simulink model "Rec3_P3_TwoLinkArm"  (R2024b)
settings: Solver=VariableStepAuto  StartTime=0.0  StopTime=10.0  RelTol=1e-3
values from neighbouring files (symbols this model uses):
  A = (1-f)/0.005    (= 50)    [Rec3_P3_TwoLinkArm_Triangle_script.m]    (also in Rec_5_main.m)
  f = 0.75    [Rec3_P3_TwoLinkArm_Triangle_script.m]    (also in Rec_5_main.m)
  Kd1 = 1.6169    [Rec3_P3_TwoLinkArm_Triangle_script.m]    (also in Rec_5_main.m)
  Kd2 = Kd1    (= 1.6169)    [Rec3_P3_TwoLinkArm_Triangle_script.m]    (also in Rec_5_main.m)
  Kp1 = 11.4196    [Rec3_P3_TwoLinkArm_Triangle_script.m]    (also in Rec_5_main.m)
  Kp2 = Kp1    (= 11.4196)    [Rec3_P3_TwoLinkArm_Triangle_script.m]    (also in Rec_5_main.m)
  sim_t = [linspace(0,8,4*n)]    [Rec3_P3_TwoLinkArm_Triangle_script.m]
  theta_1_sim = zeros(1,length(sim_t))    [Rec3_P3_TwoLinkArm_Triangle_script.m]
  theta_2_sim = zeros(1,length(sim_t))    [Rec3_P3_TwoLinkArm_Triangle_script.m]
settings Model: Creator=tibbe
settings SolverCC: AlgebraicLoopSolver=TrustRegion
settings DataIOCC: ReturnWorkspaceOutputs=off
settings OptimizationCC: ReuseModelBlockBuffer=off
settings DebuggingCC: UnconnectedInputMsg=warning  UnconnectedOutputMsg=warning  UnconnectedLineMsg=warning  ArithmeticOperatorsInVariantConditions=warning
settings ModelReferenceCC: EnableRefExpFcnMdlSchedulingChecks=on
settings SFSimCC: SimUseLocalCustomCode=off  CustomCodeUndefinedFunction=UseInterfaceOnly
settings RTWCC: RTWUseLocalCustomCode=off  GPUComputeCapability=3.5

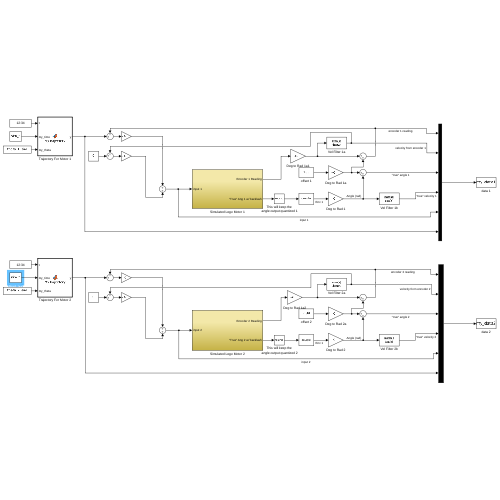
[thumbnail: Simulink's stored preview of the top-level diagram]
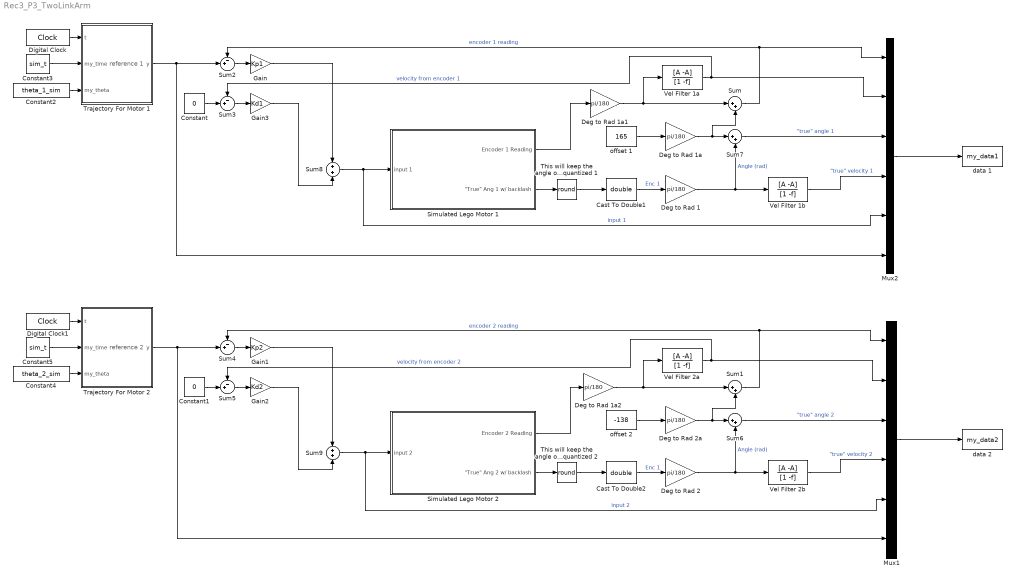
== system Rec3_P3_TwoLinkArm ==
  note: reference 1
  note: reference 2
  Cast To Double1 : DataTypeConversion  OutDataTypeStr=double  SaturateOnIntegerOverflow=off  RndMeth=Floor
  Cast To Double2 : DataTypeConversion  OutDataTypeStr=double  SaturateOnIntegerOverflow=off  RndMeth=Floor
  Constant : Constant  Value=0
  Constant1 : Constant  Value=0
  Constant2 : Constant  Value=theta_1_sim
  Constant3 : Constant  Value=sim_t
  Constant4 : Constant  Value=theta_2_sim
  Constant5 : Constant  Value=sim_t
  Deg to Rad 1 : Gain  Gain=pi/180
  Deg to Rad 1a : Gain  Gain=pi/180
  Deg to Rad 1a1 : Gain  Gain=pi/180
  Deg to Rad 1a2 : Gain  Gain=pi/180
  Deg to Rad 2 : Gain  Gain=pi/180
  Deg to Rad 2a : Gain  Gain=pi/180
  Digital Clock : DigitalClock  SampleTime=5e-3
  Digital Clock1 : DigitalClock  SampleTime=5e-3
  Gain : Gain  Gain=Kp1
  Gain1 : Gain  Gain=Kp2
  Gain2 : Gain  Gain=Kd2
  Gain3 : Gain  Gain=Kd1
  Mux1 : Mux  Inputs=6
  Mux2 : Mux  Inputs=6
  Simulated Lego Motor 1 : Subsystem
  Simulated Lego Motor 2 : Subsystem
  Sum{,1,6..7} (4 alike) : Sum  Inputs=|++
  Sum{2..5} (4 alike) : Sum  Inputs=-+|
  Sum8 : Sum
  Sum9 : Sum
  This will keep the angle output quantized 1 : Rounding  Operator=round
  This will keep the angle output quantized 2 : Rounding  Operator=round
  Trajectory For Motor 1 : MATLAB Function  TreatAsAtomicUnit=on
  Trajectory For Motor 2 : MATLAB Function  TreatAsAtomicUnit=on
  Vel Filter 1a : DiscreteTransferFcn  Numerator=[A -A]  Denominator=[1 -f]
  Vel Filter 1b : DiscreteTransferFcn  Numerator=[A -A]  Denominator=[1 -f]
  Vel Filter 2a : DiscreteTransferFcn  Numerator=[A -A]  Denominator=[1 -f]
  Vel Filter 2b : DiscreteTransferFcn  Numerator=[A -A]  Denominator=[1 -f]
  data 1 : ToWorkspace  VariableName=my_data1  SaveFormat=Structure With Time  SampleTime=-1
  data 2 : ToWorkspace  VariableName=my_data2  SaveFormat=Structure With Time  SampleTime=-1
  offset 1 : Constant  Value=165
  offset 2 : Constant  Value=-138
  wires:
  Simulated Lego Motor 1/2("\"True\" Ang 1 w/ backlash") -> This will keep the angle output quantized 1/1
  offset 1/1 -> Deg to Rad 1a/1
  Deg to Rad 1/1 -> Sum7/2, Vel Filter 1b/1  "Angle (rad)"
  Cast To Double1/1 -> Deg to Rad 1/1  "Enc 1"
  Deg to Rad 1a/1 -> Sum7/1, Sum/2
  This will keep the angle output quantized 1/1 -> Cast To Double1/1
  Sum7/1 -> Mux2/3  "\"true\" angle 1"
  Mux2/1 -> data 1/1
  Simulated Lego Motor 1/1(Encoder 1 Reading) -> Deg to Rad 1a1/1
  Sum/1 -> Sum2/1, Mux2/1  "encoder 1 reading"
  Sum2/1 -> Gain/1
  Sum3/1 -> Gain3/1
  Constant/1 -> Sum3/2
  Vel Filter 1b/1 -> Mux2/4  "\"true\" velocity 1"
  Vel Filter 1a/1 -> Mux2/2, Sum3/1  "velocity from encoder 1"
  This will keep the angle output quantized 2/1 -> Cast To Double2/1
  Simulated Lego Motor 2/1(Encoder 2 Reading) -> Deg to Rad 1a2/1
  Constant1/1 -> Sum5/2
  Deg to Rad 2a/1 -> Sum6/1, Sum1/2
  Trajectory For Motor 2/1(y) -> Sum4/2, Mux1/6
  Sum5/1 -> Gain2/1
  Sum6/1 -> Mux1/3  "\"true\" angle 2"
  Cast To Double2/1 -> Deg to Rad 2/1  "Enc 1"
  Deg to Rad 2/1 -> Sum6/2, Vel Filter 2b/1  "Angle (rad)"
  Sum4/1 -> Gain1/1
  Mux1/1 -> data 2/1
  Vel Filter 2a/1 -> Mux1/2, Sum5/1  "velocity from encoder 2"
  Sum1/1 -> Sum4/1, Mux1/1  "encoder 2 reading"
  Simulated Lego Motor 2/2("\"True\" Ang 2 w/ backlash") -> This will keep the angle output quantized 2/1
  offset 2/1 -> Deg to Rad 2a/1
  Vel Filter 2b/1 -> Mux1/4  "\"true\" velocity 2"
  Sum8/1 -> Simulated Lego Motor 1/1(input 1), Mux2/5  "input 1"
  Gain3/1 -> Sum8/2
  Gain/1 -> Sum8/1
  Sum9/1 -> Simulated Lego Motor 2/1(input 2), Mux1/5  "input 2"
  Gain2/1 -> Sum9/2
  Gain1/1 -> Sum9/1
  Trajectory For Motor 1/1(y) -> Mux2/6, Sum2/2
  Deg to Rad 1a1/1 -> Vel Filter 1a/1, Sum/1
  Deg to Rad 1a2/1 -> Vel Filter 2a/1, Sum1/1
  Digital Clock/1 -> Trajectory For Motor 1/1(t)
  Constant3/1 -> Trajectory For Motor 1/2(my_time)
  Constant2/1 -> Trajectory For Motor 1/3(my_theta)
  Digital Clock1/1 -> Trajectory For Motor 2/1(t)
  Constant5/1 -> Trajectory For Motor 2/2(my_time)
  Constant4/1 -> Trajectory For Motor 2/3(my_theta)

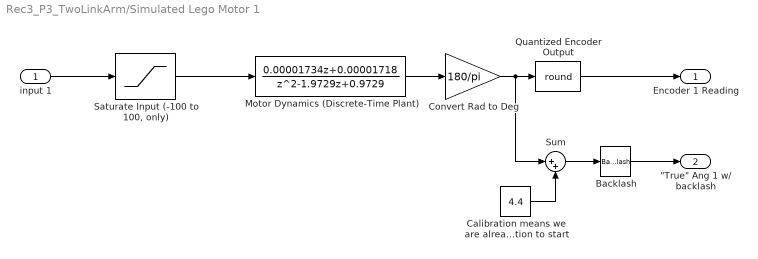
== system Rec3_P3_TwoLinkArm/Simulated Lego Motor 1 ==
  input 1 : Inport
  Backlash : Backlash  BacklashWidth=9
  "Calibration means we are already at one edge. Motor 1 calibrated in positive direction, so we push the backlash in the positive direction to start" : Constant  Value=4.4
  Convert Rad to Deg : Gain  Gain=180/pi
  Motor Dynamics (Discrete-Time Plant) : DiscreteTransferFcn  Numerator="[0.00001734  0.00001718]"  Denominator="[1   -1.9729    0.9729]"
  Quantized Encoder Output : Rounding  Operator=round
  "Saturate Input (-100 to 100, only)" : Saturate  UpperLimit=100  LowerLimit=-100
  Sum : Sum  Inputs=|++
  Encoder 1 Reading : Outport
  "\"True\" Ang 1 w/ backlash" : Outport  Port=2
  wires:
  Quantized Encoder Output/1 -> Encoder 1 Reading/1
  Motor Dynamics (Discrete-Time Plant)/1 -> Convert Rad to Deg/1
  Convert Rad to Deg/1 -> Sum/1, Quantized Encoder Output/1
  input 1/1 -> "Saturate Input (-100 to 100, only)"/1
  Backlash/1 -> "\"True\" Ang 1 w/ backlash"/1
  Sum/1 -> Backlash/1
  "Calibration means we are already at one edge. Motor 1 calibrated in positive direction, so we push the backlash in the positive direction to start"/1 -> Sum/2
  "Saturate Input (-100 to 100, only)"/1 -> Motor Dynamics (Discrete-Time Plant)/1

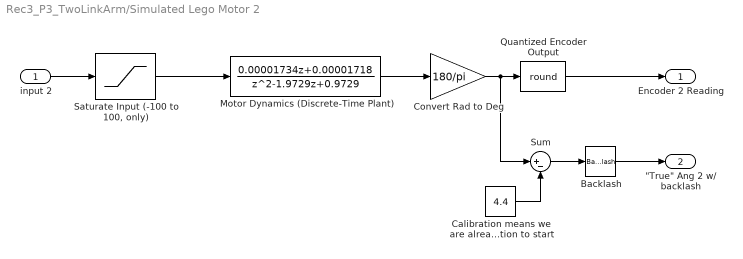
== system Rec3_P3_TwoLinkArm/Simulated Lego Motor 2 ==
  input 2 : Inport
  Backlash : Backlash  BacklashWidth=9
  "Calibration means we are already at one edge. Motor 2 calibrated in negative direction, so we push the backlash in the negative direction to start" : Constant  Value=4.4
  Convert Rad to Deg : Gain  Gain=180/pi
  Motor Dynamics (Discrete-Time Plant) : DiscreteTransferFcn  Numerator="[0.00001734  0.00001718]"  Denominator="[1   -1.9729    0.9729]"
  Quantized Encoder Output : Rounding  Operator=round
  "Saturate Input (-100 to 100, only)" : Saturate  UpperLimit=100  LowerLimit=-100
  Sum : Sum  Inputs=|+-
  Encoder 2 Reading : Outport
  "\"True\" Ang 2 w/ backlash" : Outport  Port=2
  wires:
  Quantized Encoder Output/1 -> Encoder 2 Reading/1
  Motor Dynamics (Discrete-Time Plant)/1 -> Convert Rad to Deg/1
  Convert Rad to Deg/1 -> Sum/1, Quantized Encoder Output/1
  input 2/1 -> "Saturate Input (-100 to 100, only)"/1
  Backlash/1 -> "\"True\" Ang 2 w/ backlash"/1
  Sum/1 -> Backlash/1
  "Calibration means we are already at one edge. Motor 2 calibrated in negative direction, so we push the backlash in the negative direction to start"/1 -> Sum/2
  "Saturate Input (-100 to 100, only)"/1 -> Motor Dynamics (Discrete-Time Plant)/1

== matlab function Rec3_P3_TwoLinkArm/Trajectory For Motor 2 ==
  data: t input; y output; my_time input; my_theta input
function  y  = MyTrajectory(t,my_time,my_theta)

% Define y(t) as a desired TRAJECTORY as a function of TIME

if t < my_time(1)
    % start position
    y = my_theta(1);
elseif t > my_time(end)
        y = my_theta(end);
else
    if 0
        % Example 1: step between vertices
        idx = find(t<my_time,1,'first');
        y = my_theta(idx(1));
        
    else
        % Example 2: Interpolate between given point
            y = interp1(my_time,my_theta,t);  % LINEAR INTERPOLATION, as a REFERENCE
    end
end
end

== matlab function Rec3_P3_TwoLinkArm/Trajectory For Motor 1 ==
  data: t input; y output; my_time input; my_theta input
function  y  = MyTrajectory(t,my_time,my_theta)

% Define y(t) as a desired TRAJECTORY as a function of TIME

if t < my_time(1)
    % start position
    y = my_theta(1);
elseif t > my_time(end)
        y = my_theta(end);
else
    if 0
        % Example 1: step between vertices
        idx = find(t<my_time,1,'first');
        y = my_theta(idx(1));
        
    else
        % Example 2: Interpolate between given point
            y = interp1(my_time,my_theta,t);  % LINEAR INTERPOLATION, as a REFERENCE
    end
end
end
